simulink model "calcDesTanRoll_cl_th"  (R2020a)
settings: Solver=VariableStepAuto  StartTime=0.0  StopTime=10.0  RelTol=1e-3
undefined symbols (not defined in the file or in its folder): f_kitePos, f_kiteVel, netWingLift
libraries: calcDesTanRoll_cl x1
settings Model: Creator=Ayaz  LastModifiedBy=Ayaz

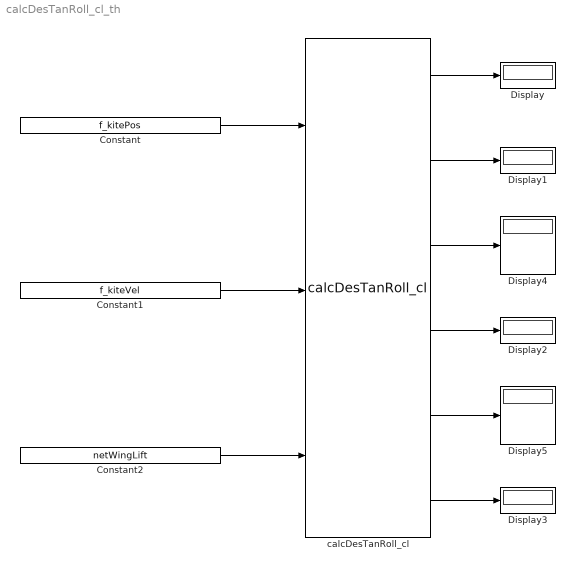
== system calcDesTanRoll_cl_th ==
  Constant : Constant  Value=f_kitePos  VectorParams1D=off
  Constant1 : Constant  Value=f_kiteVel
  Constant2 : Constant  Value=netWingLift  VectorParams1D=off
  Display{,1..5} (6 alike) : Display
  calcDesTanRoll_cl : calcDesTanRoll_cl/calcDesTanRoll_cl  fltC=fltCtrller
  wires:
  Constant/1 -> calcDesTanRoll_cl/1
  Constant1/1 -> calcDesTanRoll_cl/2
  Constant2/1 -> calcDesTanRoll_cl/3
  calcDesTanRoll_cl/1 -> Display/1
  calcDesTanRoll_cl/2 -> Display1/1
  calcDesTanRoll_cl/4 -> Display2/1
  calcDesTanRoll_cl/6 -> Display3/1
  calcDesTanRoll_cl/3 -> Display4/1
  calcDesTanRoll_cl/5 -> Display5/1
